simulink model "MicrogridExample"  (R2022b)
settings: Solver=FixedStepAuto  StartTime=0.0  StopTime=10.0  FixedStep=Ts  RelTol=1e-3
undefined symbols (not defined in the file): DCHigh, DCLow, DiscIntNeverNeededParam
libraries: fl_lib x20, nesl_utility x14
settings Model: DataDictionary=BusSystem.sldd  Creator=Finn  LastModifiedBy=cfn2169
settings SolverCC: AlgebraicLoopSolver=TrustRegion
settings DebuggingCC: UnconnectedInputMsg=warning  UnconnectedOutputMsg=warning  UnconnectedLineMsg=warning  SFMachineParentedDataDiag=warning
settings HardwareCC: TargetBitPerPointer=64  TargetBitPerSizeT=64  TargetBitPerPtrDiffT=64  TargetLongLongMode=on  TargetIntDivRoundTo=Zero  TargetEndianess=LittleEndian  TargetWordSize=64  TargetHWDeviceType=MATLAB Host  ProdEqTarget=off
settings ModelReferenceCC: EnableRefExpFcnMdlSchedulingChecks=on
settings RTWCC: Description=S-Function Target  SystemTargetFile=rtwsfcn.tlc  TemplateMakefile=rtwsfcn_default_tmf  RetainRTWFile=on  DLArmComputeVersion=19.05
settings STFCustomTargetCC: TargetLangStandard=C99 (ISO)  ModelReferenceCompliant=off  CompOptLevelCompliant=on  MATLABClassNameForMDSCustomization=Simulink.SoftwareTarget.TargetSpecificTriggerConfigurationBase  GRTInterface=on  SystemTargetFile=rtwsfcn.tlc

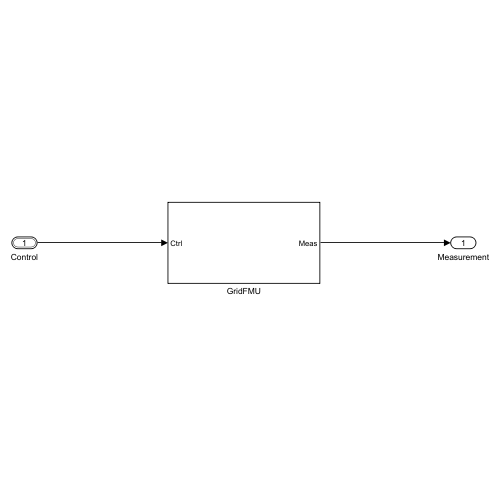
[thumbnail: Simulink's stored preview of the top-level diagram]
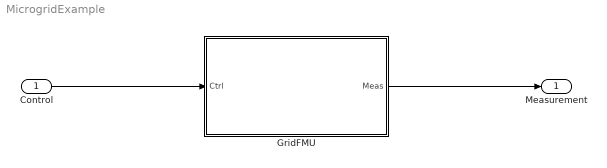
== system MicrogridExample ==
  Control : Inport  OutDataTypeStr=Bus: bus3
  GridFMU : Subsystem
  Measurement : Outport
  wires:
  Control/1 -> GridFMU/1(Ctrl)
  GridFMU/1(Meas) -> Measurement/1

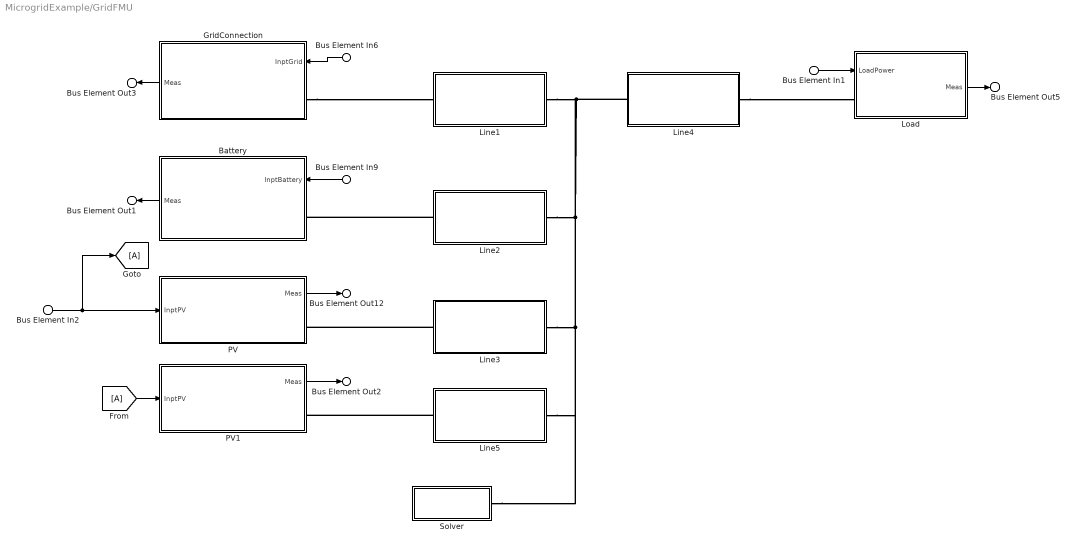
== system MicrogridExample/GridFMU ==
  Bus Element In6 : Inport  PortName=Ctrl  Element=InptGrid
  Bus Element In9 : Inport  PortName=Ctrl  Element=InptBattery
  Bus Element In1 : Inport  PortName=Ctrl  Element=InptLoad
  Bus Element In2 : Inport  PortName=Ctrl  Element=InptPV
  Battery : Subsystem  mask{Efull=4.15, Qrat=1.0, Irat=0.2, Eexp=3.7, Qexp=0.85, Enom=3.63, Qnom=0.92, Rint=0.09, Npar=5, Nser=13, T_1=1.0, Vnom=48, Droop=0.5}
      mask prompts: Efull "Fully charged voltage in V"; Qrat "Rated capacity in Ah"; Irat "Rated current in A"; Eexp "Voltage at end of exponential zone in V"; Qexp "Charge at end of exponential zone in A"; Enom "Voltage at end of nominal zone in V"; Qnom "Charge at end of nominal zone in Ah"; Rint "Internal resistance in Ohm"; Npar "Number of cells in parallel"; Nser "Number of cells in series"; T_1 "Time constant voltage control in s"; Vnom "Nominal voltage in V"; Droop "Droop coefficient in %"
      mask DialogControl DescGroupVar Prompt: Battery storage with DC/DC-Converter
      mask DialogControl DescTextVar Prompt: This model simulates in a simplified way a voltage-controlled converter for battery integration. It is modelled by a PT1-transfer function for reference changes and the droop control. The battery is modelled by a simple model with an internal resistance and a SOC-dependent voltage.
      mask DialogControl ParameterGroupVar1 Prompt: Battery parameters
      mask DialogControl ParameterGroupVar2 Prompt: Converter parameters
  From : From
  Goto : Goto
  GridConnection : Subsystem  mask{T_1=1.0, Vnom=48, Droop=0.5}
      mask prompts: T_1 "Time constant voltage control in s"; Vnom "Nominal voltage in V"; Droop "Droop coefficient in %"
      mask DialogControl DescGroupVar Prompt: Grid connection with DC/DC-Converter
      mask DialogControl DescTextVar Prompt: This model simulates in a simplified way a voltage-controlled converter for the grid connection. The voltage control is modelled by a PT1-transfer functions. Additionally, the droop control is modelled.
  Line1 : Subsystem  Description=|  mask{d=1e-3, l=15, r=1.38e-3}
      | Simple model of a wire with two conductors.
      | 
      | Resistor and Inductor of the wire are calculated based on distance and radius of the conductors and the length of the line.
      mask prompts: d "Distance between wires in m"; l "Length in m"; r "Radius of wires in m"
  Line2 : Subsystem  Description=|  mask{d=1e-3, l=10, r=1.38e-3}
      | Simple model of a wire with two conductors.
      | 
      | Resistor and Inductor of the wire are calculated based on distance and radius of the conductors and the length of the line.
      mask prompts: d "Distance between wires in m"; l "Length in m"; r "Radius of wires in m"
  Line3 : Subsystem  Description=|  mask{d=1e-3, l=10, r=1.38e-3}
      | Simple model of a wire with two conductors.
      | 
      | Resistor and Inductor of the wire are calculated based on distance and radius of the conductors and the length of the line.
      mask prompts: d "Distance between wires in m"; l "Length in m"; r "Radius of wires in m"
  Line4 : Subsystem  Description=|  mask{d=1e-3, l=10, r=1.38e-3}
      | Simple model of a wire with two conductors.
      | 
      | Resistor and Inductor of the wire are calculated based on distance and radius of the conductors and the length of the line.
      mask prompts: d "Distance between wires in m"; l "Length in m"; r "Radius of wires in m"
  Line5 : Subsystem  Description=|  mask{d=1e-3, l=10, r=1.38e-3}
      | Simple model of a wire with two conductors.
      | 
      | Resistor and Inductor of the wire are calculated based on distance and radius of the conductors and the length of the line.
      mask prompts: d "Distance between wires in m"; l "Length in m"; r "Radius of wires in m"
  Load : Subsystem  mask{Vnom=48, Slope=100, Vmin=0.8, Vmax=1.2}
      mask prompts: Vnom "Nominal Voltage in V"; Slope "Slope on/off"; Vmin "MinV relative to Vnom"; Vmax "MaxV relative to Vnom"
  PV : Subsystem  mask{A=3, eta_pv=0.2, alpha=-0.4, T_mppt=1.0}
      mask prompts: A "PV Area in m^2"; eta_pv "Efficiency PV array"; alpha "Temperature coefficient in %"; T_mppt "Time constant MPPT"
      mask DialogControl DescGroupVar Prompt: PV-Array with DC-DC-Converter
      mask DialogControl DescTextVar Prompt: This model simulates in a simplified way a converter with MPPT-control for PV integration. The reaction of the converter and its power output to an irradiance step are modelled by a PT1-transfer function. The PV-array model is based on the maximum output power at a certain irradiance and module temperature.
      mask DialogControl ParameterGroupVar1 Prompt: PV parameters
      mask DialogControl Container3 Prompt: Converter/Control parameters
  PV1 : Subsystem  mask{A=3, eta_pv=0.2, alpha=-0.4, T_mppt=1.0}
      mask prompts: A "PV Area in m^2"; eta_pv "Efficiency PV array"; alpha "Temperature coefficient in %"; T_mppt "Time constant MPPT"
      mask DialogControl DescGroupVar Prompt: PV-Array with DC-DC-Converter
      mask DialogControl DescTextVar Prompt: This model simulates in a simplified way a converter with MPPT-control for PV integration. The reaction of the converter and its power output to an irradiance step are modelled by a PT1-transfer function. The PV-array model is based on the maximum output power at a certain irradiance and module temperature.
      mask DialogControl ParameterGroupVar1 Prompt: PV parameters
      mask DialogControl Container3 Prompt: Converter/Control parameters
  Solver : Subsystem
  Bus Element Out1 : Outport  PortName=Meas  Element=Battery
  Bus Element Out5 : Outport  PortName=Meas  Element=Load
  Bus Element Out3 : Outport  PortName=Meas  Element=Grid
  Bus Element Out12 : Outport  PortName=Meas  Element=PV
  Bus Element Out2 : Outport  PortName=Meas  Element=PV1
  wires:
  Battery/1(Meas) -> Bus Element Out1/1
  Load/1(Meas) -> Bus Element Out5/1
  Bus Element In1/1 -> Load/1(LoadPower)
  GridConnection/1(Meas) -> Bus Element Out3/1
  Bus Element In9/1 -> Battery/1(InptBattery)
  PV/1(Meas) -> Bus Element Out12/1
  Bus Element In6/1 -> GridConnection/1(InptGrid)
  Bus Element In2/1 -> Goto/1, PV/1(InptPV)
  PV1/1(Meas) -> Bus Element Out2/1
  From/1 -> PV1/1(InptPV)
  connections:
  Line1/RConn1 -- Solver/RConn1 -- Line5/RConn1 -- Line3/RConn1 -- Line2/RConn1 -- Line4/LConn1
  Line4/RConn1 -- Load/LConn1
  GridConnection/LConn1 -- Line1/LConn1
  Line2/LConn1 -- Battery/LConn1
  Line3/LConn1 -- PV/RConn1
  Line5/LConn1 -- PV1/RConn1

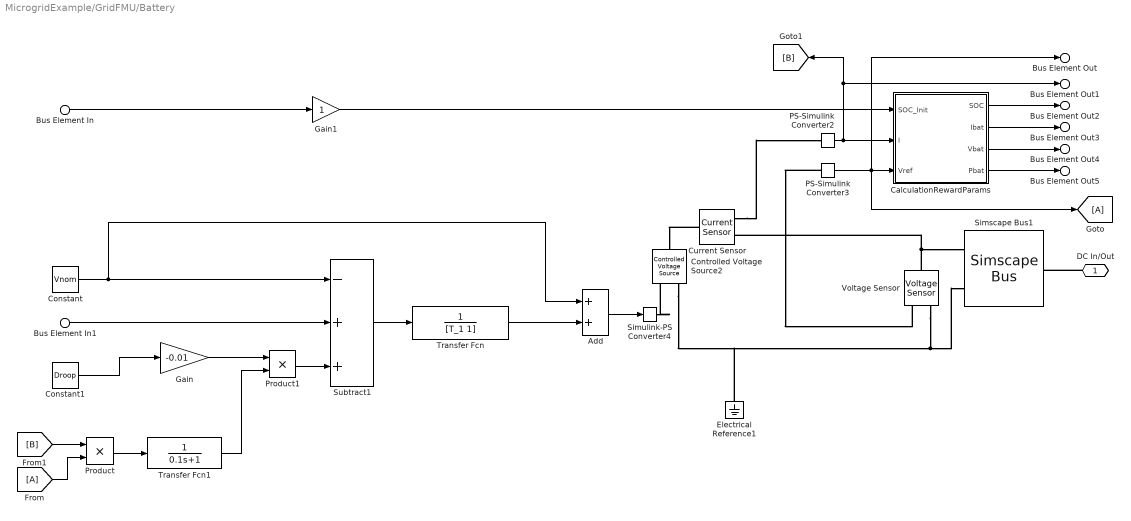
== system MicrogridExample/GridFMU/Battery ==
  Bus Element In : Inport  PortName=InptBattery  Element=SOC_Init
  Bus Element In1 : Inport  PortName=InptBattery  Element=VoltageReference
  Add : Sum
  CalculationRewardParams : Subsystem  mask{Efull=Efull, Qrat=Qrat, Irat=Irat, Eexp=Eexp, Qexp=Qexp, Enom=Enom, Qnom=Qnom, Rint=Rint, Npar=Npar, Nser=Nser}
      mask prompts: Efull "Fully charged voltage in V"; Qrat "Rated capacity in Ah"; Irat "Rated current in A"; Eexp "Voltage at end of exponential zone in V"; Qexp "Charge at end of exponential zone in AH"; Enom "Voltage at end of nominal zone in V"; Qnom "Charge at end of nominal zone in Ah"; Rint "Internal resistance in Ohm"; Npar "Number of cells in parallel"; Nser "Number of cells in series"
  Constant : Constant  Value=Vnom
  Constant1 : Constant  Value=Droop
  Controlled Voltage Source2 : fl_lib/Electrical/Electrical Sources/Controlled Voltage Source
  Current Sensor : fl_lib/Electrical/Electrical Sensors/Current Sensor
  Electrical Reference1 : fl_lib/Electrical/Electrical Elements/Electrical Reference
  From : From
  Gain : Gain  Gain=-0.01
  Gain1 : Gain
  Goto : Goto
  PS-Simulink Converter2 : nesl_utility/PS-Simulink Converter  PhysicalDomain=network_engine_domain  SubClassName=ps_output  LeftPortType=input  RightPortType=output  PseudoPeriodic=off  Frequencies=[]  VectorFormat=1-D array  Unit=inherit  AffineConversion=off
  PS-Simulink Converter3 : nesl_utility/PS-Simulink Converter  PhysicalDomain=network_engine_domain  SubClassName=ps_output  LeftPortType=input  RightPortType=output  PseudoPeriodic=off  Frequencies=[]  VectorFormat=1-D array  Unit=inherit  AffineConversion=off
  Product : Product
  Product1 : Product
  Simscape Bus1 : SimscapeBus  HierarchyStrings=DCHigh;DCLow
  Simulink-PS Converter4 : nesl_utility/Simulink-PS Converter  PhysicalDomain=network_engine_domain  SubClassName=ps_input  LeftPortType=input  RightPortType=output  PseudoPeriodic=off  Frequencies=[]  NoiseDistribution=none  NoiseParameters=[]  Unit=1  AffineConversion=off  FilteringAndDerivatives=provide  SimscapeFilterOrder=1  InputFilterTimeConstant=0.001  UdotUserProvided=0
  Subtract1 : Sum  Inputs=-++
  Transfer Fcn : TransferFcn  Denominator=[T_1 1]
  Transfer Fcn1 : TransferFcn  Denominator=[0.1 1]
  Voltage Sensor : fl_lib/Electrical/Electrical Sensors/Voltage Sensor
  DC In/Out : PMIOPort  Side=Left
  Bus Element Out : Outport  PortName=Meas  Element=Vnet
  Bus Element Out1 : Outport  PortName=Meas  Element=Inet
  Bus Element Out2 : Outport  PortName=Meas  Element=SOC
  Bus Element Out3 : Outport  PortName=Meas  Element=Ibat
  Bus Element Out4 : Outport  PortName=Meas  Element=Vbat
  Bus Element Out5 : Outport  PortName=Meas  Element=Pbat
  wires:
  PS-Simulink Converter2/1 -> CalculationRewardParams/2(I), [B], Bus Element Out1/1
  CalculationRewardParams/1(SOC) -> Bus Element Out2/1
  CalculationRewardParams/2(Ibat) -> Bus Element Out3/1
  PS-Simulink Converter3/1 -> CalculationRewardParams/3(Vref), Bus Element Out/1, Goto/1
  CalculationRewardParams/4(Pbat) -> Bus Element Out5/1
  CalculationRewardParams/3(Vbat) -> Bus Element Out4/1
  Gain/1 -> Product1/1
  Bus Element In/1 -> Gain1/1
  Constant1/1 -> Gain/1
  Transfer Fcn1/1 -> Product1/2
  Product/1 -> Transfer Fcn1/1
  Product1/1 -> Subtract1/3
  Transfer Fcn/1 -> Add/2
  From/1 -> Product/2
  Constant/1 -> Add/1, Subtract1/1
  [B] -> Product/1
  Add/1 -> Simulink-PS Converter4/1
  Subtract1/1 -> Transfer Fcn/1
  Bus Element In1/1 -> Subtract1/2
  Gain1/1 -> CalculationRewardParams/1(SOC_Init)
  connections:
  Voltage Sensor/LConn1 -- Current Sensor/RConn2 -- Simscape Bus1/LConn1
  Voltage Sensor/RConn2 -- Simscape Bus1/LConn2 -- Controlled Voltage Source2/RConn2 -- Electrical Reference1/LConn1
  PS-Simulink Converter3/LConn1 -- Voltage Sensor/RConn1
  Current Sensor/LConn1 -- Controlled Voltage Source2/LConn1
  DC In/Out/RConn1 -- Simscape Bus1/RConn1
  Simulink-PS Converter4/RConn1 -- Controlled Voltage Source2/RConn1
  Current Sensor/RConn1 -- PS-Simulink Converter2/LConn1

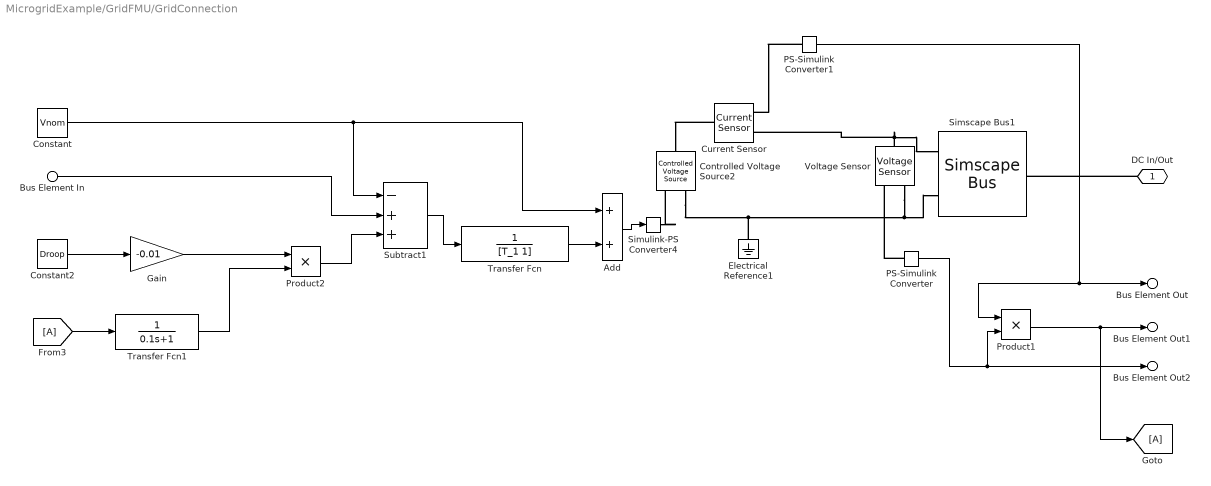
== system MicrogridExample/GridFMU/GridConnection ==
  Bus Element In : Inport  PortName=InptGrid  Element=VoltageReference
  Add : Sum
  Constant : Constant  Value=Vnom
  Constant2 : Constant  Value=Droop
  Controlled Voltage Source2 : fl_lib/Electrical/Electrical Sources/Controlled Voltage Source
  Current Sensor : fl_lib/Electrical/Electrical Sensors/Current Sensor
  Electrical Reference1 : fl_lib/Electrical/Electrical Elements/Electrical Reference
  From3 : From
  Gain : Gain  Gain=-0.01
  Goto : Goto
  PS-Simulink Converter : nesl_utility/PS-Simulink Converter  PhysicalDomain=network_engine_domain  SubClassName=ps_output  LeftPortType=input  RightPortType=output  PseudoPeriodic=off  Frequencies=[]  VectorFormat=1-D array  Unit=inherit  AffineConversion=off
  PS-Simulink Converter1 : nesl_utility/PS-Simulink Converter  PhysicalDomain=network_engine_domain  SubClassName=ps_output  LeftPortType=input  RightPortType=output  PseudoPeriodic=off  Frequencies=[]  VectorFormat=1-D array  Unit=inherit  AffineConversion=off
  Product1 : Product
  Product2 : Product
  Simscape Bus1 : SimscapeBus  HierarchyStrings=DCHigh;DCLow
  Simulink-PS Converter4 : nesl_utility/Simulink-PS Converter  PhysicalDomain=network_engine_domain  SubClassName=ps_input  LeftPortType=input  RightPortType=output  PseudoPeriodic=off  Frequencies=[]  NoiseDistribution=none  NoiseParameters=[]  Unit=1  AffineConversion=off  FilteringAndDerivatives=provide  SimscapeFilterOrder=1  InputFilterTimeConstant=0.001  UdotUserProvided=0
  Subtract1 : Sum  Inputs=-++
  Transfer Fcn : TransferFcn  Denominator=[T_1 1]
  Transfer Fcn1 : TransferFcn  Denominator=[0.1 1]
  Voltage Sensor : fl_lib/Electrical/Electrical Sensors/Voltage Sensor
  DC In/Out : PMIOPort  Side=Left
  Bus Element Out : Outport  PortName=Meas  Element=I
  Bus Element Out1 : Outport  PortName=Meas  Element=P
  Bus Element Out2 : Outport  PortName=Meas  Element=V
  wires:
  Bus Element In/1 -> Subtract1/2
  PS-Simulink Converter/1 -> Bus Element Out2/1, Product1/2
  Product1/1 -> Goto/1, Bus Element Out1/1
  Product2/1 -> Subtract1/3
  Subtract1/1 -> Transfer Fcn/1
  Constant/1 -> Add/1, Subtract1/1
  Add/1 -> Simulink-PS Converter4/1
  Gain/1 -> Product2/1
  Transfer Fcn1/1 -> Product2/2
  Constant2/1 -> Gain/1
  From3/1 -> Transfer Fcn1/1
  Transfer Fcn/1 -> Add/2
  PS-Simulink Converter1/1 -> Product1/1, Bus Element Out/1
  connections:
  Voltage Sensor/RConn2 -- Electrical Reference1/LConn1 -- Controlled Voltage Source2/RConn2 -- Simscape Bus1/LConn2
  Current Sensor/RConn2 -- Simscape Bus1/LConn1 -- Voltage Sensor/LConn1
  DC In/Out/RConn1 -- Simscape Bus1/RConn1
  PS-Simulink Converter/LConn1 -- Voltage Sensor/RConn1
  PS-Simulink Converter1/LConn1 -- Current Sensor/RConn1
  Simulink-PS Converter4/RConn1 -- Controlled Voltage Source2/RConn1
  Current Sensor/LConn1 -- Controlled Voltage Source2/LConn1

== system MicrogridExample/GridFMU/Line1 ==
  Simscape Component : SimscapeComponentBlock  SourceFile=Wire_2Cond  ComponentPath=Wire_2Cond  ComponentVariants="[\"Wire_2Cond\"]"  ComponentVariantNames="[\"Wire_2Cond\"]"  ClassName=Wire_2Cond  SchemaVersion=1  d=d  L=l  r=r  specR=1.68e-8 Ohm  Lh_specify=off  Lh_priority=None  Lh=0 A  Lh_nominal_specify=off  Lh_nominal_unit=A  Lh_nominal_value=1  Ll_specify=off  Ll_priority=None  Ll=0 A  Ll_nominal_specify=off  Ll_nominal_unit=A  Ll_nominal_value=1
      settings: CopyFcn=simscape.engine.sli.internal.componentblockcallback(gcbh,'COPY')  PreCopyFcn=simscape.engine.sli.internal.componentblockcallback(gcbh,'PRECOPY')  PreDeleteFcn=simscape.engine.sli.internal.componentblockcallback(gcbh,'PREDELETE')  InternalSimscapePortConfiguration="{\"Bottom\":[],\"Left\":[{\"id\":\"hIn\",\"label\":\"Hin\",\"type\":\"foundation.electrical.electrical\"},{\"id\":\"lIn\",\"label\":\"Lin\",\"type\":\"foundation.electrical.electrical\"}],\"Right\":[{\"id\":\"hOut\",\"label\":\"Hout\",\"type\":\"foundation.electrical.electrical\"},{\"id\":\"lOut\",\"label\":\"Lout\",\"type\":\"foundation.electrical.electrical\"}],\"Top\":[]}"
      mask Type: wire2 Conductors
  Simscape Bus1 : SimscapeBus  HierarchyStrings=DCHigh;DCLow
  Simscape Bus2 : SimscapeBus  HierarchyStrings=DCHigh;DCLow
  DC Out : PMIOPort  Side=Right
  DC In : PMIOPort  Port=2  Side=Left
  connections:
  Simscape Bus1/RConn1 -- DC Out/RConn1
  Simscape Bus1/LConn1 -- Simscape Component/RConn1
  Simscape Component/LConn1 -- Simscape Bus2/LConn1
  Simscape Bus2/LConn2 -- Simscape Component/LConn2
  DC In/RConn1 -- Simscape Bus2/RConn1
  Simscape Component/RConn2 -- Simscape Bus1/LConn2

== system MicrogridExample/GridFMU/Line2 ==
  Simscape Component : SimscapeComponentBlock  SourceFile=Wire_2Cond  ComponentPath=Wire_2Cond  ComponentVariants="[\"Wire_2Cond\"]"  ComponentVariantNames="[\"Wire_2Cond\"]"  ClassName=Wire_2Cond  SchemaVersion=1  d=d  L=l  r=r  specR=1.68e-8 Ohm  Lh_specify=off  Lh_priority=None  Lh=0 A  Lh_nominal_specify=off  Lh_nominal_unit=A  Lh_nominal_value=1  Ll_specify=off  Ll_priority=None  Ll=0 A  Ll_nominal_specify=off  Ll_nominal_unit=A  Ll_nominal_value=1
      settings: CopyFcn=simscape.engine.sli.internal.componentblockcallback(gcbh,'COPY')  PreCopyFcn=simscape.engine.sli.internal.componentblockcallback(gcbh,'PRECOPY')  PreDeleteFcn=simscape.engine.sli.internal.componentblockcallback(gcbh,'PREDELETE')  InternalSimscapePortConfiguration="{\"Bottom\":[],\"Left\":[{\"id\":\"hIn\",\"label\":\"Hin\",\"type\":\"foundation.electrical.electrical\"},{\"id\":\"lIn\",\"label\":\"Lin\",\"type\":\"foundation.electrical.electrical\"}],\"Right\":[{\"id\":\"hOut\",\"label\":\"Hout\",\"type\":\"foundation.electrical.electrical\"},{\"id\":\"lOut\",\"label\":\"Lout\",\"type\":\"foundation.electrical.electrical\"}],\"Top\":[]}"
      mask Type: wire2 Conductors
  Simscape Bus1 : SimscapeBus  HierarchyStrings=DCHigh;DCLow
  Simscape Bus2 : SimscapeBus  HierarchyStrings=DCHigh;DCLow
  DC Out : PMIOPort  Side=Right
  DC In : PMIOPort  Port=2  Side=Left
  connections:
  Simscape Bus1/RConn1 -- DC Out/RConn1
  Simscape Bus1/LConn1 -- Simscape Component/RConn1
  Simscape Component/LConn1 -- Simscape Bus2/LConn1
  Simscape Bus2/LConn2 -- Simscape Component/LConn2
  DC In/RConn1 -- Simscape Bus2/RConn1
  Simscape Component/RConn2 -- Simscape Bus1/LConn2

== system MicrogridExample/GridFMU/Line3 ==
  Simscape Component : SimscapeComponentBlock  SourceFile=Wire_2Cond  ComponentPath=Wire_2Cond  ComponentVariants="[\"Wire_2Cond\"]"  ComponentVariantNames="[\"Wire_2Cond\"]"  ClassName=Wire_2Cond  SchemaVersion=1  d=d  L=l  r=r  specR=1.68e-8 Ohm  Lh_specify=off  Lh_priority=None  Lh=0 A  Lh_nominal_specify=off  Lh_nominal_unit=A  Lh_nominal_value=1  Ll_specify=off  Ll_priority=None  Ll=0 A  Ll_nominal_specify=off  Ll_nominal_unit=A  Ll_nominal_value=1
      settings: CopyFcn=simscape.engine.sli.internal.componentblockcallback(gcbh,'COPY')  PreCopyFcn=simscape.engine.sli.internal.componentblockcallback(gcbh,'PRECOPY')  PreDeleteFcn=simscape.engine.sli.internal.componentblockcallback(gcbh,'PREDELETE')  InternalSimscapePortConfiguration="{\"Bottom\":[],\"Left\":[{\"id\":\"hIn\",\"label\":\"Hin\",\"type\":\"foundation.electrical.electrical\"},{\"id\":\"lIn\",\"label\":\"Lin\",\"type\":\"foundation.electrical.electrical\"}],\"Right\":[{\"id\":\"hOut\",\"label\":\"Hout\",\"type\":\"foundation.electrical.electrical\"},{\"id\":\"lOut\",\"label\":\"Lout\",\"type\":\"foundation.electrical.electrical\"}],\"Top\":[]}"
      mask Type: wire2 Conductors
  Simscape Bus1 : SimscapeBus  HierarchyStrings=DCHigh;DCLow
  Simscape Bus2 : SimscapeBus  HierarchyStrings=DCHigh;DCLow
  DC Out : PMIOPort  Side=Right
  DC In : PMIOPort  Port=2  Side=Left
  connections:
  Simscape Bus1/RConn1 -- DC Out/RConn1
  Simscape Bus1/LConn1 -- Simscape Component/RConn1
  Simscape Component/LConn1 -- Simscape Bus2/LConn1
  Simscape Bus2/LConn2 -- Simscape Component/LConn2
  DC In/RConn1 -- Simscape Bus2/RConn1
  Simscape Component/RConn2 -- Simscape Bus1/LConn2

== system MicrogridExample/GridFMU/Line4 ==
  Simscape Component : SimscapeComponentBlock  SourceFile=Wire_2Cond  ComponentPath=Wire_2Cond  ComponentVariants="[\"Wire_2Cond\"]"  ComponentVariantNames="[\"Wire_2Cond\"]"  ClassName=Wire_2Cond  SchemaVersion=1  d=d  L=l  r=r  specR=1.68e-8 Ohm  Lh_specify=off  Lh_priority=None  Lh=0 A  Lh_nominal_specify=off  Lh_nominal_unit=A  Lh_nominal_value=1  Ll_specify=off  Ll_priority=None  Ll=0 A  Ll_nominal_specify=off  Ll_nominal_unit=A  Ll_nominal_value=1
      settings: CopyFcn=simscape.engine.sli.internal.componentblockcallback(gcbh,'COPY')  PreCopyFcn=simscape.engine.sli.internal.componentblockcallback(gcbh,'PRECOPY')  PreDeleteFcn=simscape.engine.sli.internal.componentblockcallback(gcbh,'PREDELETE')  InternalSimscapePortConfiguration="{\"Bottom\":[],\"Left\":[{\"id\":\"hIn\",\"label\":\"Hin\",\"type\":\"foundation.electrical.electrical\"},{\"id\":\"lIn\",\"label\":\"Lin\",\"type\":\"foundation.electrical.electrical\"}],\"Right\":[{\"id\":\"hOut\",\"label\":\"Hout\",\"type\":\"foundation.electrical.electrical\"},{\"id\":\"lOut\",\"label\":\"Lout\",\"type\":\"foundation.electrical.electrical\"}],\"Top\":[]}"
      mask Type: wire2 Conductors
  Simscape Bus1 : SimscapeBus  HierarchyStrings=DCHigh;DCLow
  Simscape Bus2 : SimscapeBus  HierarchyStrings=DCHigh;DCLow
  DC Out : PMIOPort  Side=Right
  DC In : PMIOPort  Port=2  Side=Left
  connections:
  Simscape Bus1/RConn1 -- DC Out/RConn1
  Simscape Bus1/LConn1 -- Simscape Component/RConn1
  Simscape Component/LConn1 -- Simscape Bus2/LConn1
  Simscape Bus2/LConn2 -- Simscape Component/LConn2
  DC In/RConn1 -- Simscape Bus2/RConn1
  Simscape Component/RConn2 -- Simscape Bus1/LConn2

== system MicrogridExample/GridFMU/Line5 ==
  Simscape Component : SimscapeComponentBlock  SourceFile=Wire_2Cond  ComponentPath=Wire_2Cond  ComponentVariants="[\"Wire_2Cond\"]"  ComponentVariantNames="[\"Wire_2Cond\"]"  ClassName=Wire_2Cond  SchemaVersion=1  d=d  L=l  r=r  specR=1.68e-8 Ohm  Lh_specify=off  Lh_priority=None  Lh=0 A  Lh_nominal_specify=off  Lh_nominal_unit=A  Lh_nominal_value=1  Ll_specify=off  Ll_priority=None  Ll=0 A  Ll_nominal_specify=off  Ll_nominal_unit=A  Ll_nominal_value=1
      settings: CopyFcn=simscape.engine.sli.internal.componentblockcallback(gcbh,'COPY')  PreCopyFcn=simscape.engine.sli.internal.componentblockcallback(gcbh,'PRECOPY')  PreDeleteFcn=simscape.engine.sli.internal.componentblockcallback(gcbh,'PREDELETE')  InternalSimscapePortConfiguration="{\"Bottom\":[],\"Left\":[{\"id\":\"hIn\",\"label\":\"Hin\",\"type\":\"foundation.electrical.electrical\"},{\"id\":\"lIn\",\"label\":\"Lin\",\"type\":\"foundation.electrical.electrical\"}],\"Right\":[{\"id\":\"hOut\",\"label\":\"Hout\",\"type\":\"foundation.electrical.electrical\"},{\"id\":\"lOut\",\"label\":\"Lout\",\"type\":\"foundation.electrical.electrical\"}],\"Top\":[]}"
      mask Type: wire2 Conductors
  Simscape Bus1 : SimscapeBus  HierarchyStrings=DCHigh;DCLow
  Simscape Bus2 : SimscapeBus  HierarchyStrings=DCHigh;DCLow
  DC Out : PMIOPort  Side=Right
  DC In : PMIOPort  Port=2  Side=Left
  connections:
  Simscape Bus1/RConn1 -- DC Out/RConn1
  Simscape Bus1/LConn1 -- Simscape Component/RConn1
  Simscape Component/LConn1 -- Simscape Bus2/LConn1
  Simscape Bus2/LConn2 -- Simscape Component/LConn2
  DC In/RConn1 -- Simscape Bus2/RConn1
  Simscape Component/RConn2 -- Simscape Bus1/LConn2

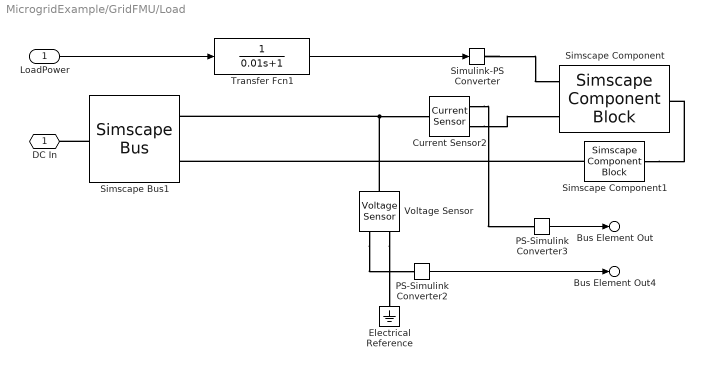
== system MicrogridExample/GridFMU/Load ==
  LoadPower : Inport
  Current Sensor2 : fl_lib/Electrical/Electrical Sensors/Current Sensor
  Electrical Reference : fl_lib/Electrical/Electrical Elements/Electrical Reference
  PS-Simulink Converter2 : nesl_utility/PS-Simulink Converter  PhysicalDomain=network_engine_domain  SubClassName=ps_output  LeftPortType=input  RightPortType=output  PseudoPeriodic=off  Frequencies=[]  VectorFormat=1-D array  Unit=inherit  AffineConversion=off
  PS-Simulink Converter3 : nesl_utility/PS-Simulink Converter  PhysicalDomain=network_engine_domain  SubClassName=ps_output  LeftPortType=input  RightPortType=output  PseudoPeriodic=off  Frequencies=[]  VectorFormat=1-D array  Unit=inherit  AffineConversion=off
  Simscape Component : SimscapeComponentBlock  SourceFile=VariablePowerLoad  ComponentPath=VariablePowerLoad  ComponentVariants="[\"VariablePowerLoad\"]"  ComponentVariantNames="[\"VariablePowerLoad\"]"  ClassName=VariablePowerLoad  SchemaVersion=1  Vsoll=Vnom  Slope=Slope  MinV=Vmin  MaxV=Vmax  i_specify=off  i_priority=None  i=0 A  i_nominal_specify=off  i_nominal_unit=A  i_nominal_value=1  v_specify=off  v_priority=None  v=0 V  v_nominal_specify=off  v_nominal_unit=V  v_nominal_value=1  Psoll_specify=off  Psoll_priority=None  Psoll=0 W  Psoll_nominal_specify=off  Psoll_nominal_unit=W  Psoll_nominal_value=1
      settings: CopyFcn=simscape.engine.sli.internal.componentblockcallback(gcbh,'COPY')  PreCopyFcn=simscape.engine.sli.internal.componentblockcallback(gcbh,'PRECOPY')  PreDeleteFcn=simscape.engine.sli.internal.componentblockcallback(gcbh,'PREDELETE')  InternalSimscapePortConfiguration="{\"Bottom\":[],\"Left\":[{\"id\":\"Power\",\"label\":\"P\",\"type\":\"input\"},{\"id\":\"p\",\"label\":\"+\",\"type\":\"foundation.electrical.electrical\"}],\"Right\":[{\"id\":\"n\",\"label\":\"-\",\"type\":\"foundation.electrical.electrical\"}],\"Top\":[]}"
      mask Type: Variable power load. It might be necesarry to use local simscape solver.
  Simscape Component1 : SimscapeComponentBlock  SourceFile=shortCircuit  ComponentPath=shortCircuit  ComponentVariants="[\"shortCircuit\"]"  ComponentVariantNames="[\"shortCircuit\"]"  ClassName=shortCircuit  SchemaVersion=1
      settings: CopyFcn=simscape.engine.sli.internal.componentblockcallback(gcbh,'COPY')  PreCopyFcn=simscape.engine.sli.internal.componentblockcallback(gcbh,'PRECOPY')  PreDeleteFcn=simscape.engine.sli.internal.componentblockcallback(gcbh,'PREDELETE')  InternalSimscapePortConfiguration="{\"Bottom\":[],\"Left\":[{\"id\":\"p\",\"label\":\"+\",\"type\":\"foundation.electrical.electrical\"}],\"Right\":[{\"id\":\"n\",\"label\":\"-\",\"type\":\"foundation.electrical.electrical\"}],\"Top\":[]}"
      mask Type: shortCircuit
  Simscape Bus1 : SimscapeBus  HierarchyStrings=DCHigh;DCLow
  Simulink-PS Converter : nesl_utility/Simulink-PS Converter  PhysicalDomain=network_engine_domain  SubClassName=ps_input  LeftPortType=input  RightPortType=output  PseudoPeriodic=off  Frequencies=[]  NoiseDistribution=none  NoiseParameters=[]  Unit=1  AffineConversion=off  FilteringAndDerivatives=provide  SimscapeFilterOrder=1  InputFilterTimeConstant=0.001  UdotUserProvided=0
  Transfer Fcn1 : TransferFcn  Denominator=[0.01 1]
  Voltage Sensor : fl_lib/Electrical/Electrical Sensors/Voltage Sensor
  DC In : PMIOPort  Side=Left
  Bus Element Out : Outport  PortName=Meas  Element=I
  Bus Element Out4 : Outport  PortName=Meas  Element=V
  wires:
  PS-Simulink Converter3/1 -> Bus Element Out/1
  LoadPower/1 -> Transfer Fcn1/1
  Transfer Fcn1/1 -> Simulink-PS Converter/1
  PS-Simulink Converter2/1 -> Bus Element Out4/1
  connections:
  Simscape Component1/RConn1 -- Simscape Bus1/LConn2
  Voltage Sensor/LConn1 -- Current Sensor2/LConn1 -- Simscape Bus1/LConn1
  Voltage Sensor/RConn1 -- PS-Simulink Converter2/LConn1
  Simulink-PS Converter/RConn1 -- Simscape Component/LConn1
  Simscape Component1/LConn1 -- Simscape Component/RConn1
  Simscape Bus1/RConn1 -- DC In/RConn1
  Current Sensor2/RConn2 -- Simscape Component/LConn2
  Current Sensor2/RConn1 -- PS-Simulink Converter3/LConn1
  Voltage Sensor/RConn2 -- Electrical Reference/LConn1

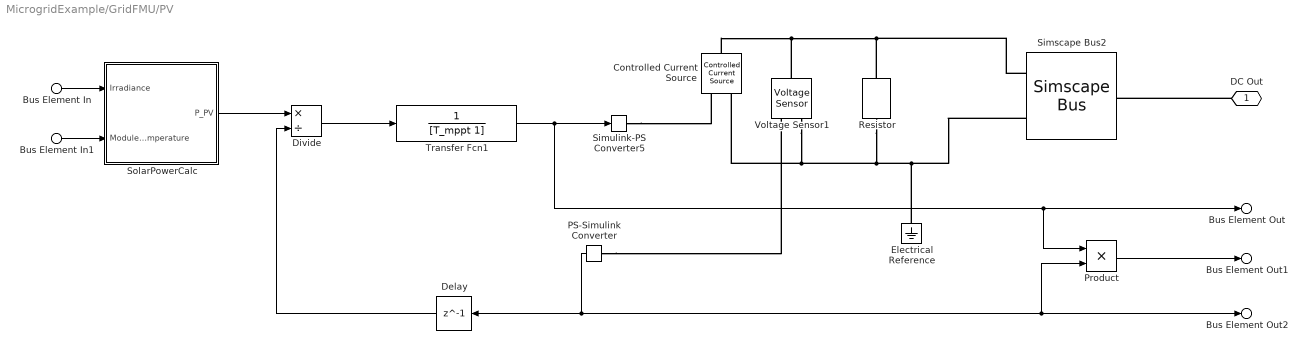
== system MicrogridExample/GridFMU/PV ==
  Bus Element In : Inport  PortName=InptPV  Element=Irradiance
  Bus Element In1 : Inport  PortName=InptPV  Element=ModuleTemperature
  Controlled Current Source : fl_lib/Electrical/Electrical Sources/Controlled Current Source
  Delay : Delay  DelayLength=1  InitialCondition=48.0
  Divide : Product  Inputs=*/
  Electrical Reference : fl_lib/Electrical/Electrical Elements/Electrical Reference
  PS-Simulink Converter : nesl_utility/PS-Simulink Converter  PhysicalDomain=network_engine_domain  SubClassName=ps_output  LeftPortType=input  RightPortType=output  PseudoPeriodic=off  Frequencies=[]  VectorFormat=1-D array  Unit=inherit  AffineConversion=off
  Product : Product
  Resistor : fl_lib/Electrical/Electrical Elements/Resistor  R=1e9 Ohm  i_specify=off  i_priority=None  i=0 A  i_nominal_specify=off  i_nominal_unit=A  i_nominal_value=1  v_specify=off  v_priority=None  v=0 V  v_nominal_specify=off  v_nominal_unit=V  v_nominal_value=1
  Simscape Bus2 : SimscapeBus  HierarchyStrings=DCHigh;DCLow
  Simulink-PS Converter5 : nesl_utility/Simulink-PS Converter  PhysicalDomain=network_engine_domain  SubClassName=ps_input  LeftPortType=input  RightPortType=output  PseudoPeriodic=off  Frequencies=[]  NoiseDistribution=none  NoiseParameters=[]  Unit=1  AffineConversion=off  FilteringAndDerivatives=provide  SimscapeFilterOrder=1  InputFilterTimeConstant=0.001  UdotUserProvided=0
  SolarPowerCalc : Subsystem
  Transfer Fcn1 : TransferFcn  Denominator=[T_mppt 1]
  Voltage Sensor1 : fl_lib/Electrical/Electrical Sensors/Voltage Sensor
  DC Out : PMIOPort  Side=Right
  Bus Element Out : Outport  PortName=Meas  Element=I
  Bus Element Out1 : Outport  PortName=Meas  Element=P
  Bus Element Out2 : Outport  PortName=Meas  Element=V
  wires:
  Transfer Fcn1/1 -> Bus Element Out/1, Product/1, Simulink-PS Converter5/1
  PS-Simulink Converter/1 -> Bus Element Out2/1, Product/2, Delay/1
  Product/1 -> Bus Element Out1/1
  Bus Element In/1 -> SolarPowerCalc/1(Irradiance)
  Bus Element In1/1 -> SolarPowerCalc/2(ModuleTemperature)
  SolarPowerCalc/1(P_PV) -> Divide/1
  Divide/1 -> Transfer Fcn1/1
  Delay/1 -> Divide/2
  connections:
  Voltage Sensor1/LConn1 -- Controlled Current Source/LConn1 -- Simscape Bus2/LConn1 -- Resistor/LConn1
  Simscape Bus2/LConn2 -- Electrical Reference/LConn1 -- Controlled Current Source/RConn2 -- Voltage Sensor1/RConn2 -- Resistor/RConn1
  PS-Simulink Converter/LConn1 -- Voltage Sensor1/RConn1
  Simulink-PS Converter5/RConn1 -- Controlled Current Source/RConn1
  DC Out/RConn1 -- Simscape Bus2/RConn1

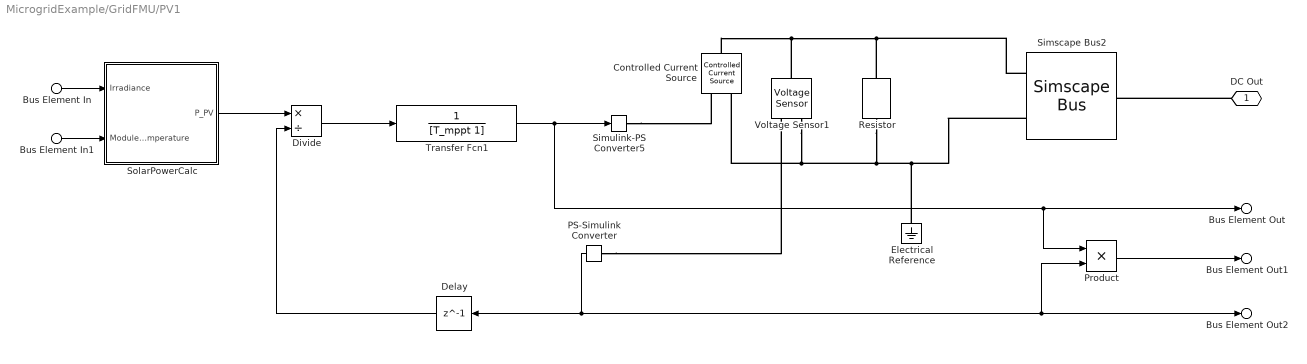
== system MicrogridExample/GridFMU/PV1 ==
  Bus Element In : Inport  PortName=InptPV  Element=Irradiance
  Bus Element In1 : Inport  PortName=InptPV  Element=ModuleTemperature
  Controlled Current Source : fl_lib/Electrical/Electrical Sources/Controlled Current Source
  Delay : Delay  DelayLength=1  InitialCondition=48.0
  Divide : Product  Inputs=*/
  Electrical Reference : fl_lib/Electrical/Electrical Elements/Electrical Reference
  PS-Simulink Converter : nesl_utility/PS-Simulink Converter  PhysicalDomain=network_engine_domain  SubClassName=ps_output  LeftPortType=input  RightPortType=output  PseudoPeriodic=off  Frequencies=[]  VectorFormat=1-D array  Unit=inherit  AffineConversion=off
  Product : Product
  Resistor : fl_lib/Electrical/Electrical Elements/Resistor  R=1e9 Ohm  i_specify=off  i_priority=None  i=0 A  i_nominal_specify=off  i_nominal_unit=A  i_nominal_value=1  v_specify=off  v_priority=None  v=0 V  v_nominal_specify=off  v_nominal_unit=V  v_nominal_value=1
  Simscape Bus2 : SimscapeBus  HierarchyStrings=DCHigh;DCLow
  Simulink-PS Converter5 : nesl_utility/Simulink-PS Converter  PhysicalDomain=network_engine_domain  SubClassName=ps_input  LeftPortType=input  RightPortType=output  PseudoPeriodic=off  Frequencies=[]  NoiseDistribution=none  NoiseParameters=[]  Unit=1  AffineConversion=off  FilteringAndDerivatives=provide  SimscapeFilterOrder=1  InputFilterTimeConstant=0.001  UdotUserProvided=0
  SolarPowerCalc : Subsystem
  Transfer Fcn1 : TransferFcn  Denominator=[T_mppt 1]
  Voltage Sensor1 : fl_lib/Electrical/Electrical Sensors/Voltage Sensor
  DC Out : PMIOPort  Side=Right
  Bus Element Out : Outport  PortName=Meas  Element=I
  Bus Element Out1 : Outport  PortName=Meas  Element=P
  Bus Element Out2 : Outport  PortName=Meas  Element=V
  wires:
  Transfer Fcn1/1 -> Bus Element Out/1, Product/1, Simulink-PS Converter5/1
  PS-Simulink Converter/1 -> Bus Element Out2/1, Product/2, Delay/1
  Product/1 -> Bus Element Out1/1
  Bus Element In/1 -> SolarPowerCalc/1(Irradiance)
  Bus Element In1/1 -> SolarPowerCalc/2(ModuleTemperature)
  SolarPowerCalc/1(P_PV) -> Divide/1
  Divide/1 -> Transfer Fcn1/1
  Delay/1 -> Divide/2
  connections:
  Voltage Sensor1/LConn1 -- Controlled Current Source/LConn1 -- Simscape Bus2/LConn1 -- Resistor/LConn1
  Simscape Bus2/LConn2 -- Electrical Reference/LConn1 -- Controlled Current Source/RConn2 -- Voltage Sensor1/RConn2 -- Resistor/RConn1
  PS-Simulink Converter/LConn1 -- Voltage Sensor1/RConn1
  Simulink-PS Converter5/RConn1 -- Controlled Current Source/RConn1
  DC Out/RConn1 -- Simscape Bus2/RConn1

== system MicrogridExample/GridFMU/Solver ==
  Electrical Reference : fl_lib/Electrical/Electrical Elements/Electrical Reference
  Simscape Bus2 : SimscapeBus  HierarchyStrings=DCHigh;DCLow
  Solver Configuration : nesl_utility/Solver Configuration  PhysicalDomain=network_engine_domain  SubClassName=solver  LeftPortType=input  RightPortType=generic  Tones=[]  Harmonics=[]  SimulateNoise=off  Profile=off  UseLocalSampling=off  EnableSwitchedLinearOptims=on  FrequencyDomain=off  UseCCode=off  RelTol=0.001  AbsTol=1e-06  MinStep=1e-09  ToWorkspace=off  RevertToSquareIcSolve=off  NumHomotopyIterations=100  PhasorMode=off  PhasorModeNumHarmonics=1  ConsistencySolver=NEWTON_FTOL  IndexReductionMethod=DerivativeReplacement  DoDC=on  ResidualTolerance=1e-09  ConsistencyTolSource=GLOBAL  ConsistencyAbsTol=0.001  ConsistencyRelTol=0.001  ConsistencyTolFactor=0.001  UseLocalSolver=on  LocalSolverChoice=NE_BACKWARD_EULER_ADVANCER  ResolveIndetEquations=on  FunctionEvalNumThread=1  LocalSolverSampleTime=Ts  DoFixedCost=on  MaxNonlinIter=3  MaxModeIter=2  ComputeImpulses=off  ImpulseIterations=2  LinearAlgebra=auto  LinearAlgebraNumThread=0  EquationFormulation=NE_TIME_EF  DelaysMemoryBudget=1024  AutomaticFiltering=off  FilteringTimeConstant=0.001  PartitionStorageMethod=AS_NEEDED  PartitionMemoryBudget=1024  PartitionMethod=ROBUST
  LVDCBus : PMIOPort  Side=Right
  connections:
  Simscape Bus2/RConn1 -- LVDCBus/RConn1
  Simscape Bus2/LConn1 -- Solver Configuration/RConn1
  Electrical Reference/LConn1 -- Simscape Bus2/LConn2

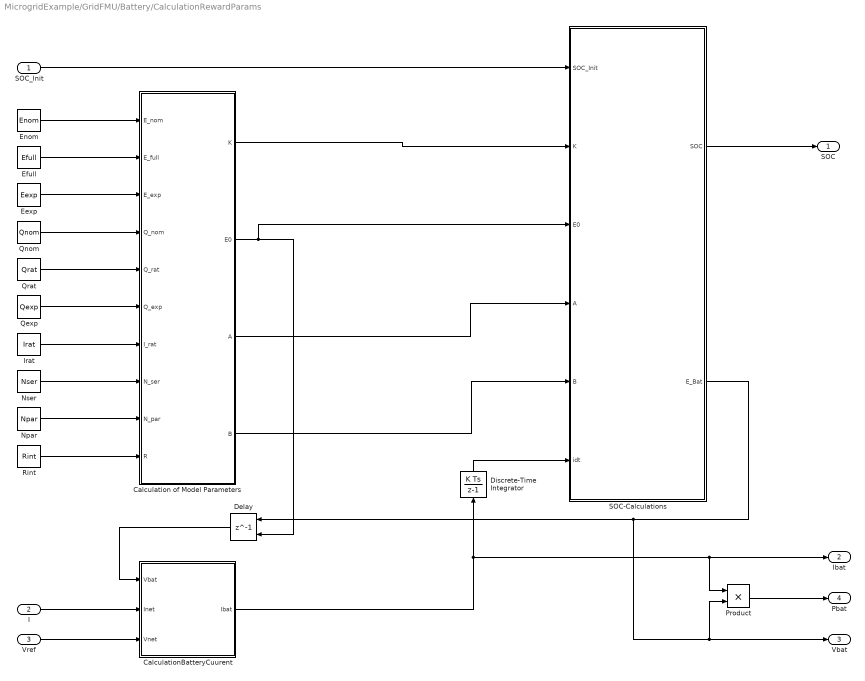
== system MicrogridExample/GridFMU/Battery/CalculationRewardParams ==
  SOC_Init : Inport
  I : Inport  Port=2
  Vref : Inport  Port=3
  Calculation of Model Parameters : Subsystem
  CalculationBatteryCuurent : Subsystem
  Delay : Delay  DelayLength=1  InitialConditionSource=Input port  InitialCondition=1
      settings: InputPortMap=u0,p4
  Discrete-Time Integrator : DiscreteIntegrator  SampleTime=-1  ICPrevOutput=DiscIntNeverNeededParam  ICPrevScaledInput=DiscIntNeverNeededParam
  Eexp : Constant  Value=Eexp
  Efull : Constant  Value=Efull
  Enom : Constant  Value=Enom
  Irat : Constant  Value=Irat
  Npar : Constant  Value=Npar
  Nser : Constant  Value=Nser
  Product : Product
  Qexp : Constant  Value=Qexp
  Qnom : Constant  Value=Qnom
  Qrat : Constant  Value=Qrat
  Rint : Constant  Value=Rint
  SOC-Calculations : Subsystem
  SOC : Outport
  Ibat : Outport  Port=2
  Vbat : Outport  Port=3
  Pbat : Outport  Port=4
  wires:
  SOC-Calculations/2(E_Bat) -> Vbat/1, Product/2, Delay/1
  Vref/1 -> CalculationBatteryCuurent/3(Vnet)
  CalculationBatteryCuurent/1(Ibat) -> Ibat/1, Product/1, Discrete-Time Integrator/1
  SOC-Calculations/1(SOC) -> SOC/1
  Delay/1 -> CalculationBatteryCuurent/1(Vbat)
  Calculation of Model Parameters/4(B) -> SOC-Calculations/5(B)
  Discrete-Time Integrator/1 -> SOC-Calculations/6(idt)
  Enom/1 -> Calculation of Model Parameters/1(E_nom)
  Calculation of Model Parameters/3(A) -> SOC-Calculations/4(A)
  SOC_Init/1 -> SOC-Calculations/1(SOC_Init)
  Irat/1 -> Calculation of Model Parameters/7(I_rat)
  Qnom/1 -> Calculation of Model Parameters/4(Q_nom)
  I/1 -> CalculationBatteryCuurent/2(Inet)
  Calculation of Model Parameters/2(E0) -> Delay/2, SOC-Calculations/3(E0)
  Product/1 -> Pbat/1
  Nser/1 -> Calculation of Model Parameters/8(N_ser)
  Qrat/1 -> Calculation of Model Parameters/5(Q_rat)
  Efull/1 -> Calculation of Model Parameters/2(E_full)
  Calculation of Model Parameters/1(K) -> SOC-Calculations/2(K)
  Qexp/1 -> Calculation of Model Parameters/6(Q_exp)
  Rint/1 -> Calculation of Model Parameters/10(R)
  Eexp/1 -> Calculation of Model Parameters/3(E_exp)
  Npar/1 -> Calculation of Model Parameters/9(N_par)

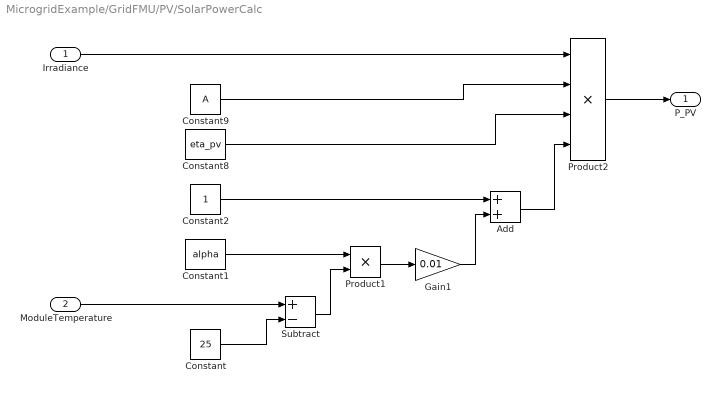
== system MicrogridExample/GridFMU/PV/SolarPowerCalc ==
  Irradiance : Inport
  ModuleTemperature : Inport  Port=2
  Add : Sum
  Constant : Constant  Value=25
  Constant1 : Constant  Value=alpha
  Constant2 : Constant
  Constant8 : Constant  Value=eta_pv
  Constant9 : Constant  Value=A
  Gain1 : Gain  Gain=0.01
  Product1 : Product
  Product2 : Product  Inputs=4
  Subtract : Sum  Inputs=+-
  P_PV : Outport
  wires:
  Product1/1 -> Gain1/1
  Constant1/1 -> Product1/1
  Constant8/1 -> Product2/3
  Constant9/1 -> Product2/2
  Constant/1 -> Subtract/2
  Add/1 -> Product2/4
  Subtract/1 -> Product1/2
  Constant2/1 -> Add/1
  Gain1/1 -> Add/2
  Irradiance/1 -> Product2/1
  ModuleTemperature/1 -> Subtract/1
  Product2/1 -> P_PV/1

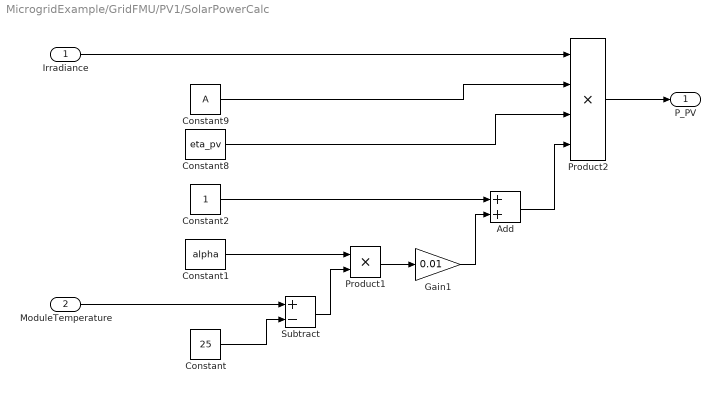
== system MicrogridExample/GridFMU/PV1/SolarPowerCalc ==
  Irradiance : Inport
  ModuleTemperature : Inport  Port=2
  Add : Sum
  Constant : Constant  Value=25
  Constant1 : Constant  Value=alpha
  Constant2 : Constant
  Constant8 : Constant  Value=eta_pv
  Constant9 : Constant  Value=A
  Gain1 : Gain  Gain=0.01
  Product1 : Product
  Product2 : Product  Inputs=4
  Subtract : Sum  Inputs=+-
  P_PV : Outport
  wires:
  Product1/1 -> Gain1/1
  Constant1/1 -> Product1/1
  Constant8/1 -> Product2/3
  Constant9/1 -> Product2/2
  Constant/1 -> Subtract/2
  Add/1 -> Product2/4
  Subtract/1 -> Product1/2
  Constant2/1 -> Add/1
  Gain1/1 -> Add/2
  Irradiance/1 -> Product2/1
  ModuleTemperature/1 -> Subtract/1
  Product2/1 -> P_PV/1

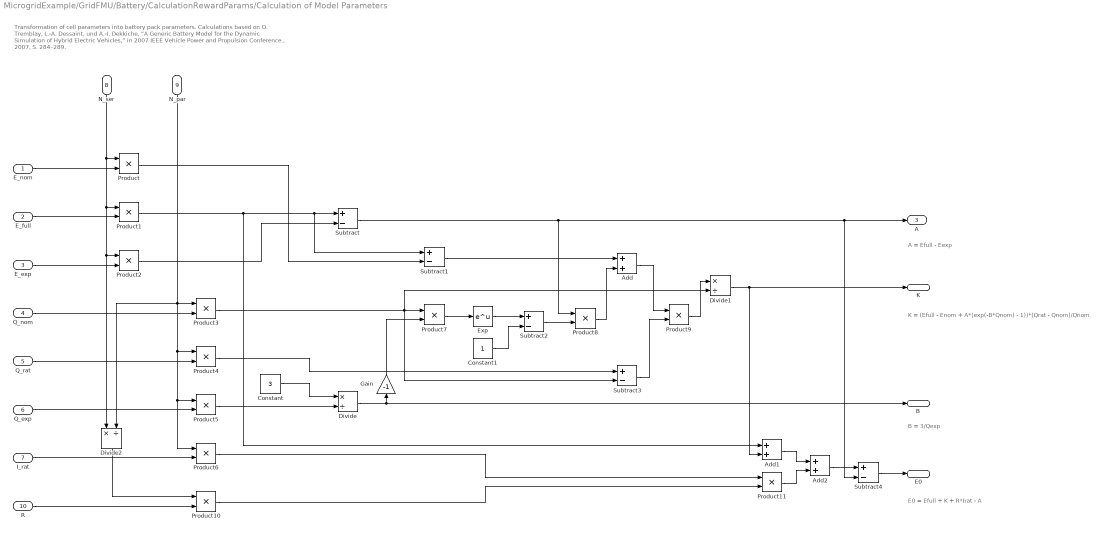
== system MicrogridExample/GridFMU/Battery/CalculationRewardParams/Calculation of Model Parameters ==
  note: Transformation of cell parameters into battery pack parameters.
      | Calculations based on O. Tremblay, L.-A. Dessaint, und A.-I. Dekkiche, “A Generic Battery Model for the Dynamic Simulation of Hybrid Electric Vehicles,” in 2007 IEEE Vehicle Power and Propulsion Conference , 2007, S. 284–289.
  note: E0 = Efull + K + R*Irat - A
  note: B = 3/Qexp
  note: K = (Efull - Enom + A*(exp(-B*Qnom) - 1))*(Qrat - Qnom)/Qnom
  note: A = Efull - Eexp
  E_nom : Inport
  E_full : Inport  Port=2
  E_exp : Inport  Port=3
  Q_nom : Inport  Port=4
  Q_rat : Inport  Port=5
  Q_exp : Inport  Port=6
  I_rat : Inport  Port=7
  N_ser : Inport  Port=8
  N_par : Inport  Port=9
  R : Inport  Port=10
  Add : Sum
  Add1 : Sum
  Add2 : Sum
  Constant : Constant  Value=3
  Constant1 : Constant
  Divide : Product  Inputs=*/
  Divide1 : Product  Inputs=*/
  Divide2 : Product  Inputs=*/
  Exp : Math
  Gain : Gain  Gain=-1
  Product{,1..11} (12 alike) : Product
  Subtract{,1..4} (5 alike) : Sum  Inputs=+-
  K : Outport
  E0 : Outport  Port=2
  A : Outport  Port=3
  B : Outport  Port=4
  wires:
  E_nom/1 -> Product/2
  N_ser/1 -> Product2/1, Divide2/1, Product1/1, Product/1
  E_full/1 -> Product1/2
  E_exp/1 -> Product2/2
  Q_nom/1 -> Product3/2
  Q_rat/1 -> Product4/2
  Q_exp/1 -> Product5/2
  N_par/1 -> Divide2/2, Product3/1, Product4/1, Product5/1, Product6/1
  I_rat/1 -> Product6/2
  Product1/1 -> Subtract/1, Subtract1/1, Add1/1
  Product2/1 -> Subtract/2
  Subtract/1 -> A/1, Subtract4/2, Product8/1
  Constant/1 -> Divide/1
  Product5/1 -> Divide/2
  Divide/1 -> B/1, Gain/1
  Product/1 -> Subtract1/2
  Gain/1 -> Product7/2
  Product3/1 -> Subtract3/2, Divide1/2, Product7/1
  Product7/1 -> Exp/1
  Subtract1/1 -> Add/1
  Exp/1 -> Subtract2/1
  Constant1/1 -> Subtract2/2
  Subtract2/1 -> Product8/2
  Product8/1 -> Add/2
  Product4/1 -> Subtract3/1
  Add/1 -> Product9/1
  Subtract3/1 -> Product9/2
  Product9/1 -> Divide1/1
  Divide1/1 -> Add1/2, K/1
  R/1 -> Product10/2
  Divide2/1 -> Product10/1
  Product6/1 -> Product11/1
  Product10/1 -> Product11/2
  Add1/1 -> Add2/1
  Product11/1 -> Add2/2
  Add2/1 -> Subtract4/1
  Subtract4/1 -> E0/1

== system MicrogridExample/GridFMU/Battery/CalculationRewardParams/CalculationBatteryCuurent ==
  Vbat : Inport
  Inet : Inport  Port=2
  Vnet : Inport  Port=3
  Add : Sum
  Constant : Constant
  Divide : Product  Inputs=*/
  Divide1 : Product  Inputs=*/
  Product2 : Product
  Subtract : Sum  Inputs=-+
  Ibat : Outport
  wires:
  Vnet/1 -> Add/1, Divide/1
  Divide/1 -> Divide1/1, Subtract/1
  Subtract/1 -> Divide1/2
  Inet/1 -> Product2/1
  Add/1 -> Divide/2
  Divide1/1 -> Product2/2
  Vbat/1 -> Add/2
  Product2/1 -> Ibat/1
  Constant/1 -> Subtract/2

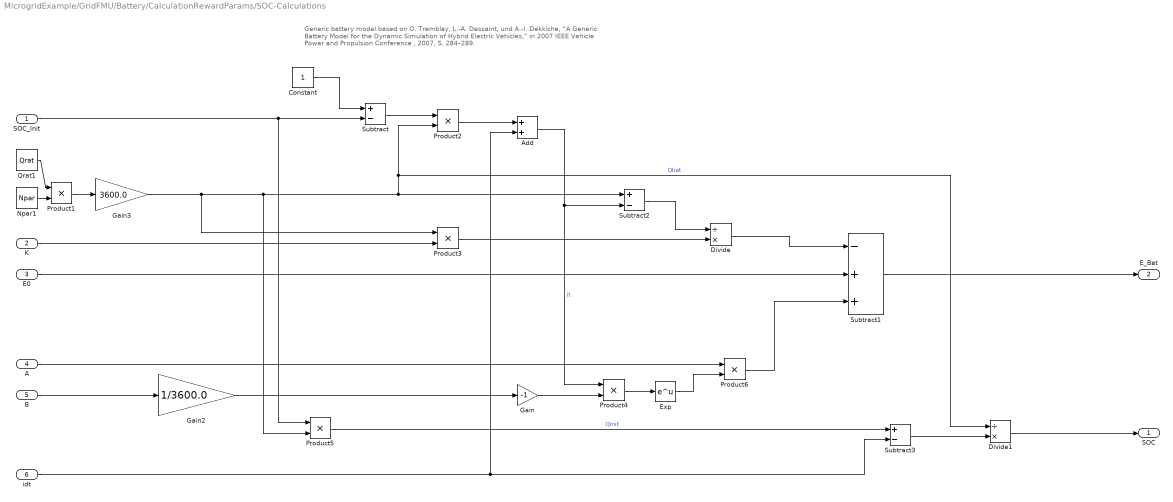
== system MicrogridExample/GridFMU/Battery/CalculationRewardParams/SOC-Calculations ==
  note: Generic battery model based on O. Tremblay, L.-A. Dessaint, und A.-I. Dekkiche, “A Generic Battery Model for the Dynamic Simulation of Hybrid Electric Vehicles,” in 2007 IEEE Vehicle Power and Propulsion Conference , 2007, S. 284–289.
  SOC_Init : Inport
  K : Inport  Port=2
  E0 : Inport  Port=3
  A : Inport  Port=4
  B : Inport  Port=5
  idt : Inport  Port=6
  Add : Sum
  Constant : Constant
  Divide : Product  Inputs=/*
  Divide1 : Product  Inputs=/*
  Exp : Math
  Gain : Gain  Gain=-1
  Gain2 : Gain  Gain=1/3600.0
  Gain3 : Gain  Gain=3600.0
  Npar1 : Constant  Value=Npar
  Product{1..6} (6 alike) : Product
  Qrat1 : Constant  Value=Qrat
  Subtract : Sum  Inputs=+-
  Subtract1 : Sum  Inputs=-++
  Subtract2 : Sum  Inputs=+-
  Subtract3 : Sum  Inputs=+-
  SOC : Outport
  E_Bat : Outport  Port=2
  wires:
  Qrat1/1 -> Product1/1
  B/1 -> Gain2/1
  SOC_Init/1 -> Subtract/2, Product5/1
  Gain/1 -> Product4/2
  Product5/1 -> Subtract3/1  "Qinit"
  idt/1 -> Add/2, Subtract3/2
  Npar1/1 -> Product1/2
  Gain2/1 -> Gain/1
  E0/1 -> Subtract1/2
  Product1/1 -> Gain3/1
  Subtract2/1 -> Divide/1
  Subtract/1 -> Product2/1
  Product2/1 -> Add/1
  Product6/1 -> Subtract1/3
  Add/1 -> Product4/1, Subtract2/2  "it"
  Product4/1 -> Exp/1
  Exp/1 -> Product6/2
  Constant/1 -> Subtract/1
  Subtract3/1 -> Divide1/2
  Product3/1 -> Divide/2
  K/1 -> Product3/2
  Divide/1 -> Subtract1/1
  Subtract1/1 -> E_Bat/1
  Divide1/1 -> SOC/1
  A/1 -> Product6/1
  Gain3/1 -> Product2/2, Divide1/1, Subtract2/1, Product5/2, Product3/1  "Qbat"
